simulink model "flow_environment_6DOF"  (R2025b)
settings: Solver=VariableStepAuto  StartTime=0.0  StopTime=10.0  RelTol=1e-3
settings Model: Creator=tmej1020  LastModifiedBy=tmej1020

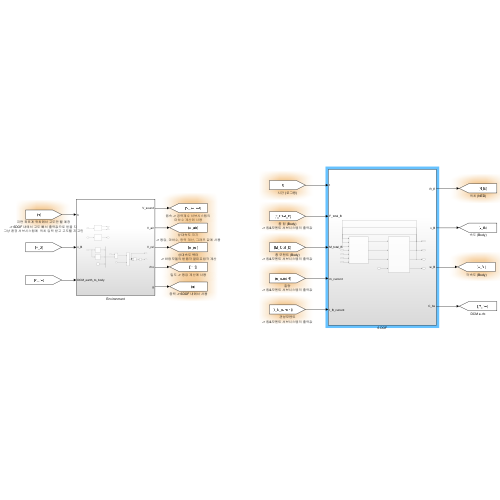
[thumbnail: Simulink's stored preview of the top-level diagram]
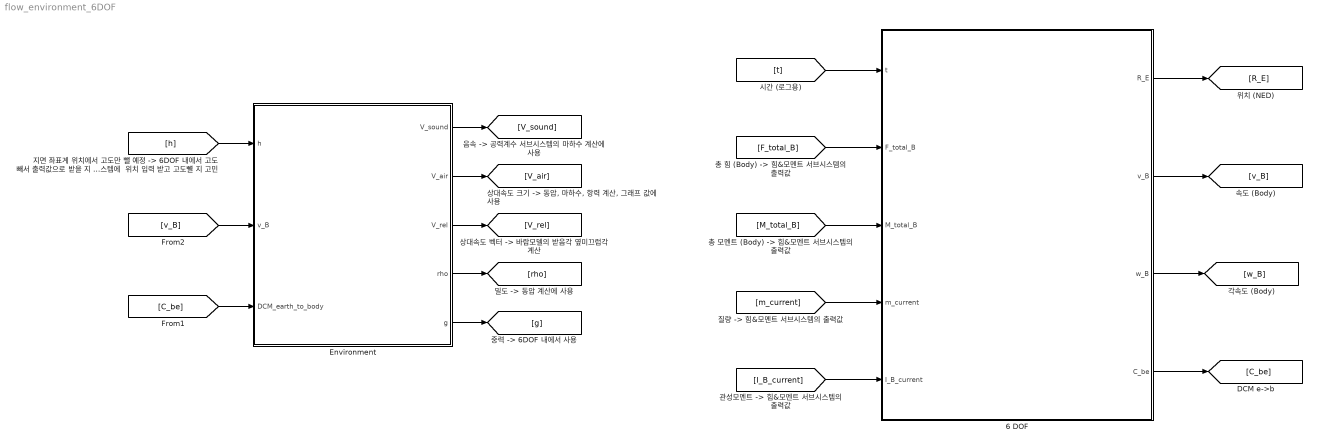
== system flow_environment_6DOF ==
  6 DOF : Subsystem
  Environment : Subsystem
  wires:
  [h] -> Environment/1(h)
  [v_B] -> Environment/2(v_B)
  [C_be] -> Environment/3(DCM_earth_to_body)
  Environment/1(V_sound) -> [V_sound]
  Environment/2(V_air) -> [V_air]
  Environment/4(rho) -> [rho]
  Environment/5(g) -> [g]
  Environment/3(V_rel) -> [V_rel]
  [t] -> 6 DOF/1(t)
  [F_total_B] -> 6 DOF/2(F_total_B)
  [M_total_B] -> 6 DOF/3(M_total_B)
  [m_current] -> 6 DOF/4(m_current)
  [I_B_current] -> 6 DOF/5(I_B_current)
  6 DOF/1(R_E) -> [R_E]
  6 DOF/2(v_B) -> [v_B]
  6 DOF/3(w_B) -> [w_B]
  6 DOF/4(C_be) -> [C_be]

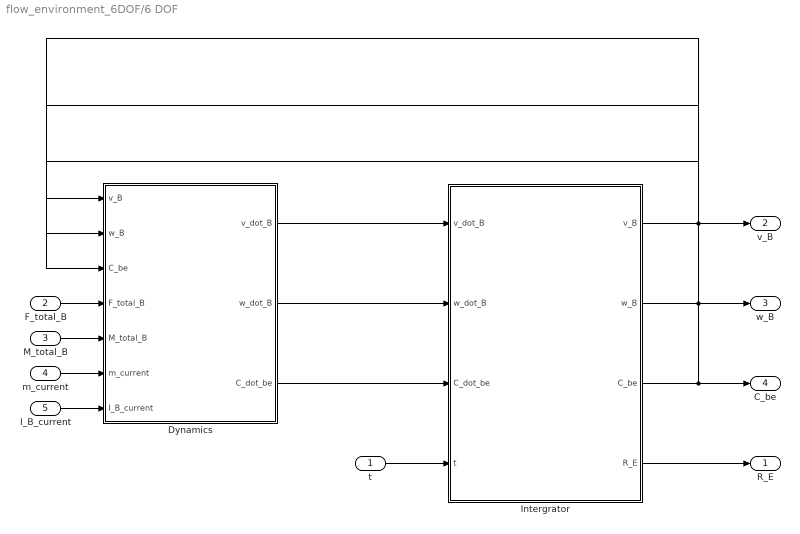
== system flow_environment_6DOF/6 DOF ==
  t : Inport
  F_total_B : Inport  Port=2
  M_total_B : Inport  Port=3
  m_current : Inport  Port=4
  I_B_current : Inport  Port=5
  Dynamics : Subsystem
  Intergrator : Subsystem
  R_E : Outport
  v_B : Outport  Port=2
  w_B : Outport  Port=3
  C_be : Outport  Port=4
  wires:
  Dynamics/1(v_dot_B) -> Intergrator/1(v_dot_B)
  Dynamics/2(w_dot_B) -> Intergrator/2(w_dot_B)
  Dynamics/3(C_dot_be) -> Intergrator/3(C_dot_be)
  t/1 -> Intergrator/4(t)
  Intergrator/1(v_B) -> Dynamics/1(v_B), v_B/1
  Intergrator/2(w_B) -> Dynamics/2(w_B), w_B/1
  Intergrator/3(C_be) -> Dynamics/3(C_be), C_be/1
  Intergrator/4(R_E) -> R_E/1
  F_total_B/1 -> Dynamics/4(F_total_B)
  M_total_B/1 -> Dynamics/5(M_total_B)
  m_current/1 -> Dynamics/6(m_current)
  I_B_current/1 -> Dynamics/7(I_B_current)

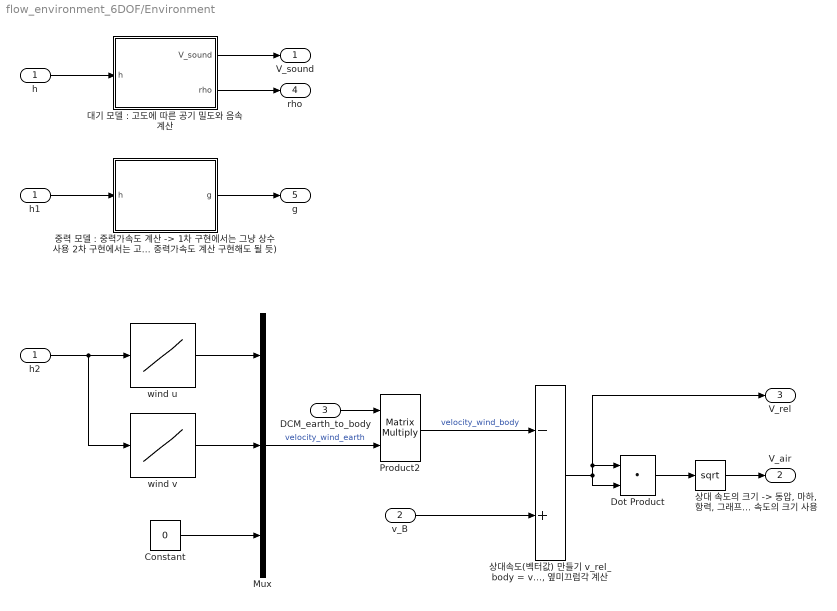
== system flow_environment_6DOF/Environment ==
  h : Inport
  v_B : Inport  Port=2
  DCM_earth_to_body : Inport  Port=3
  Constant : Constant  Value=0
  Dot Product : DotProduct  OutDataTypeStr=Inherit: Inherit via internal rule
  Mux : Mux  Inputs=3
  Product2 : Product  Multiplication=Matrix(*)
  h1 : InportShadow
  h2 : InportShadow
  wind u : Lookup_n-D  NumberOfTableDimensions=1  LookupTableObject=''  BreakpointsForDimension1=[1:2]  BreakpointsForDimension2=[1:2]  BreakpointsForDimension3=[5, 7]  BreakpointsForDimension1FirstPoint=10  BreakpointsForDimension2FirstPoint=10  BreakpointsForDimension1Spacing=12  BreakpointsForDimension2Spacing=12  IndexSearchMethod=Evenly spaced points  Table=[4 5;16 19]  InterpMethod=Flat  DiagnosticForOutOfRangeInput=Error  InternalRulePriority=Speed  RndMeth=Simplest
  wind v : Lookup_n-D  NumberOfTableDimensions=1  LookupTableObject=''  BreakpointsForDimension1=[1:2]  BreakpointsForDimension2=[1:2]  BreakpointsForDimension3=[5, 7]  BreakpointsForDimension1FirstPoint=10  BreakpointsForDimension2FirstPoint=10  BreakpointsForDimension1Spacing=12  BreakpointsForDimension2Spacing=12  IndexSearchMethod=Evenly spaced points  Table=[4 5;16 19]  InterpMethod=Flat  DiagnosticForOutOfRangeInput=Error  InternalRulePriority=Speed  RndMeth=Simplest
  "대기 모델 : 고도에 따른 공기 밀도와 음속 계산" : Subsystem
  "상대 속도의 크기 -> 동압, 마하, 항력, 그래프에는 스칼라 값인 상대 속도의 크기 사용" : Sqrt
  "상대속도(벡터값) 만들기 v_rel_body = v_body - wind_body -> 바람이 있는 경우 이 상대속도로 받음각, 옆미끄럼각 계산" : Sum  Inputs=-+
  "중력 모델 : 중력가속도 계산 -> 1차 구현에서는 그냥 상수 사용 2차 구현에서는 고도에 따른 중력가속도 계산 (근데 그냥 처음부터 고도에 따라 중력가속도 계산 구현해도 될 듯)" : Subsystem
  V_sound : Outport
  V_air : Outport  Port=2
  V_rel : Outport  Port=3
  rho : Outport  Port=4
  g : Outport  Port=5
  wires:
  h/1 -> "대기 모델 : 고도에 따른 공기 밀도와 음속 계산"/1(h)
  "대기 모델 : 고도에 따른 공기 밀도와 음속 계산"/1(V_sound) -> V_sound/1
  "대기 모델 : 고도에 따른 공기 밀도와 음속 계산"/2(rho) -> rho/1
  h1/1 -> "중력 모델 : 중력가속도 계산 -> 1차 구현에서는 그냥 상수 사용 2차 구현에서는 고도에 따른 중력가속도 계산 (근데 그냥 처음부터 고도에 따라 중력가속도 계산 구현해도 될 듯)"/1(h)
  "중력 모델 : 중력가속도 계산 -> 1차 구현에서는 그냥 상수 사용 2차 구현에서는 고도에 따른 중력가속도 계산 (근데 그냥 처음부터 고도에 따라 중력가속도 계산 구현해도 될 듯)"/1(g) -> g/1
  h2/1 -> wind u/1, wind v/1
  wind u/1 -> Mux/1
  wind v/1 -> Mux/2
  Constant/1 -> Mux/3
  Mux/1 -> Product2/2  "velocity_wind_earth"
  DCM_earth_to_body/1 -> Product2/1
  Product2/1 -> "상대속도(벡터값) 만들기 v_rel_body = v_body - wind_body -> 바람이 있는 경우 이 상대속도로 받음각, 옆미끄럼각 계산"/1  "velocity_wind_body"
  v_B/1 -> "상대속도(벡터값) 만들기 v_rel_body = v_body - wind_body -> 바람이 있는 경우 이 상대속도로 받음각, 옆미끄럼각 계산"/2
  "상대속도(벡터값) 만들기 v_rel_body = v_body - wind_body -> 바람이 있는 경우 이 상대속도로 받음각, 옆미끄럼각 계산"/1 -> Dot Product/1, V_rel/1, Dot Product/2
  Dot Product/1 -> "상대 속도의 크기 -> 동압, 마하, 항력, 그래프에는 스칼라 값인 상대 속도의 크기 사용"/1
  "상대 속도의 크기 -> 동압, 마하, 항력, 그래프에는 스칼라 값인 상대 속도의 크기 사용"/1 -> V_air/1

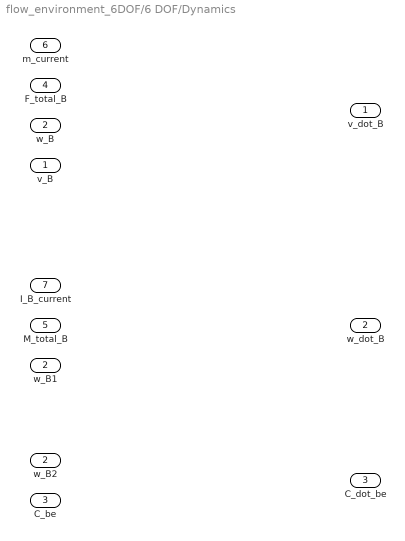
== system flow_environment_6DOF/6 DOF/Dynamics ==
  v_B : Inport
  w_B : Inport  Port=2
  C_be : Inport  Port=3
  F_total_B : Inport  Port=4
  M_total_B : Inport  Port=5
  m_current : Inport  Port=6
  I_B_current : Inport  Port=7
  w_B1 : InportShadow  Port=2
  w_B2 : InportShadow  Port=2
  v_dot_B : Outport
  w_dot_B : Outport  Port=2
  C_dot_be : Outport  Port=3

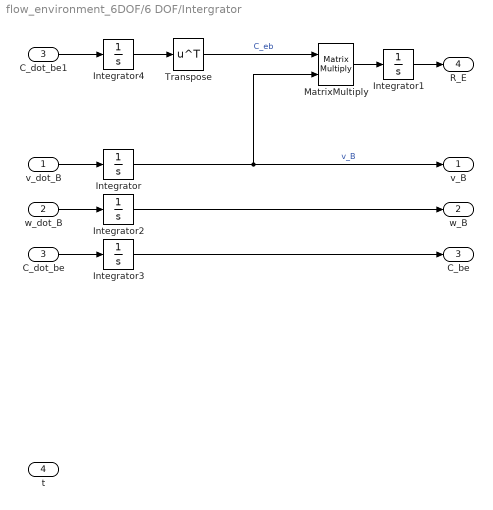
== system flow_environment_6DOF/6 DOF/Intergrator ==
  v_dot_B : Inport
  w_dot_B : Inport  Port=2
  C_dot_be : Inport  Port=3
  t : Inport  Port=4
  C_dot_be1 : InportShadow  Port=3
  Integrator{,1..4} (5 alike) : Integrator
  MatrixMultiply : Product  Multiplication=Matrix(*)
  Transpose : Math  Operator=transpose
  v_B : Outport
  w_B : Outport  Port=2
  C_be : Outport  Port=3
  R_E : Outport  Port=4
  wires:
  C_dot_be1/1 -> Integrator4/1
  v_dot_B/1 -> Integrator/1
  Integrator/1 -> MatrixMultiply/2, v_B/1  "v_B"
  MatrixMultiply/1 -> Integrator1/1
  Integrator1/1 -> R_E/1
  w_dot_B/1 -> Integrator2/1
  C_dot_be/1 -> Integrator3/1
  Integrator3/1 -> C_be/1
  Integrator2/1 -> w_B/1
  Transpose/1 -> MatrixMultiply/1  "C_eb"
  Integrator4/1 -> Transpose/1

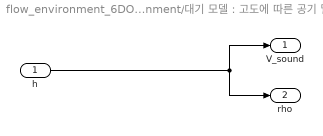
== system flow_environment_6DOF/Environment/대기 모델 : 고도에 따른 공기 밀도와 음속 계산 ==
  h : Inport
  V_sound : Outport
  rho : Outport  Port=2
  wires:
  h/1 -> V_sound/1, rho/1

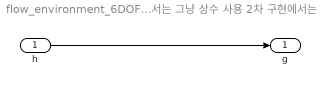
== system flow_environment_6DOF/Environment/중력 모델 : 중력가속도 계산 -> 1차 구현에서는 그냥 상수 사용 2차 구현에서는 고도에 따른 중력가속도 계산 (근데 그냥 처음부터 고도에 따라 중력가속도 계산 구현해도 될 듯) ==
  h : Inport
  g : Outport
  wires:
  h/1 -> g/1
